simulink model "Final"  (R2020b)
settings: Solver=VariableStepAuto  StartTime=0.0  StopTime=10.0  RelTol=1e-3
settings Model: Creator=Dalila  LastModifiedBy=Dalila

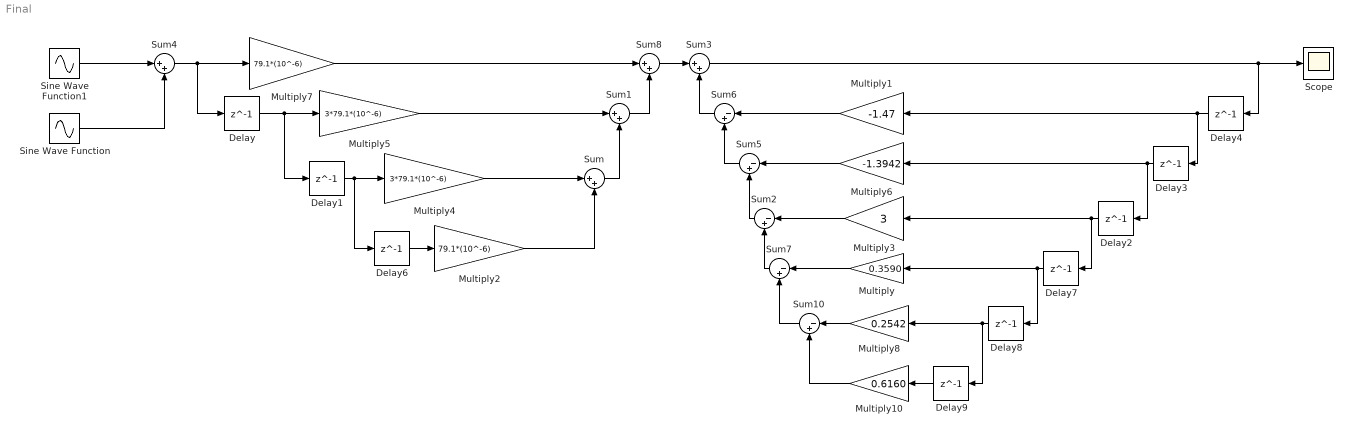
== system Final ==
  Delay{,1..4,6..9} (9 alike) : Delay  DelayLength=1  InitialCondition=0
  Multiply : Gain  Gain=0.3590
  Multiply1 : Gain  Gain=-1.47
  Multiply10 : Gain  Gain=0.6160
  Multiply2 : Gain  Gain=79.1*(10^-6)
  Multiply3 : Gain  Gain=3
  Multiply4 : Gain  Gain=3*79.1*(10^-6)
  Multiply5 : Gain  Gain=3*79.1*(10^-6)
  Multiply6 : Gain  Gain=-1.3942
  Multiply7 : Gain  Gain=79.1*(10^-6)
  Multiply8 : Gain  Gain=0.2542
  Scope : Scope
  Sine Wave Function : Sin  SineType=Sample based  Amplitude=2  Samples=5  SampleTime=0.2
  Sine Wave Function1 : Sin  SineType=Sample based  Samples=200  SampleTime=0.015
  Sum{,1,3..4,8} (5 alike) : Sum  Inputs=|++
  Sum{2,5..7,10} (5 alike) : Sum  Inputs=|-+
  wires:
  Sine Wave Function/1 -> Sum4/2
  Multiply7/1 -> Sum8/1
  Sum1/1 -> Sum8/2
  Multiply5/1 -> Sum1/1
  Delay/1 -> Delay1/1, Multiply5/1
  Delay1/1 -> Delay6/1, Multiply4/1
  Multiply4/1 -> Sum/1
  Sum/1 -> Sum1/2
  Delay6/1 -> Multiply2/1
  Sum3/1 -> Delay4/1, Scope/1
  Sum8/1 -> Sum3/1
  Sum6/1 -> Sum3/2
  Delay4/1 -> Delay3/1, Multiply1/1
  Multiply1/1 -> Sum6/1
  Delay3/1 -> Delay2/1, Multiply6/1
  Multiply6/1 -> Sum5/1
  Sum5/1 -> Sum6/2
  Delay2/1 -> Delay7/1, Multiply3/1
  Delay7/1 -> Multiply/1, Delay8/1
  Sum2/1 -> Sum5/2
  Multiply3/1 -> Sum2/1
  Multiply/1 -> Sum7/1
  Sum7/1 -> Sum2/2
  Sine Wave Function1/1 -> Sum4/1
  Sum4/1 -> Delay/1, Multiply7/1
  Multiply2/1 -> Sum/2
  Delay8/1 -> Multiply8/1, Delay9/1
  Delay9/1 -> Multiply10/1
  Sum10/1 -> Sum7/2
  Multiply8/1 -> Sum10/1
  Multiply10/1 -> Sum10/2
